simulink model "sim_model"  (R2021b)
settings: Solver=VariableStepAuto  StartTime=0.0  StopTime=10.0  RelTol=1e-3
settings Model: Creator=matteodepaola  LastModifiedBy=matteodepaola

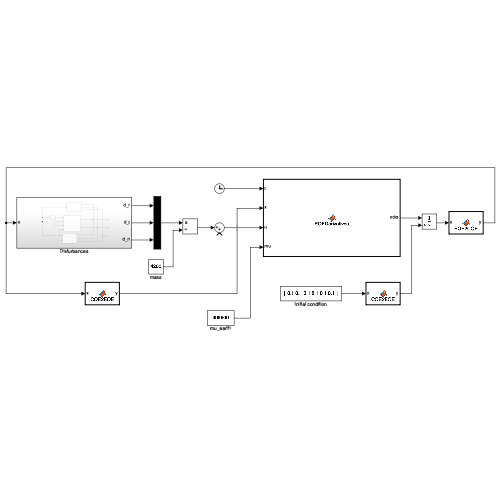
[thumbnail: Simulink's stored preview of the top-level diagram]
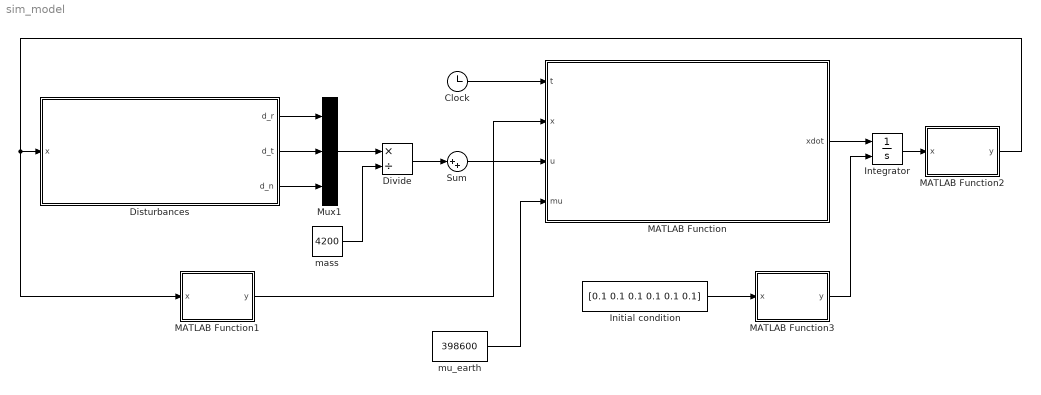
== system sim_model ==
  Clock : Clock
  Disturbances : Subsystem
  Divide : Product  Inputs=*/
  Initial condition : Constant  Value=[0.1 0.1 0.1 0.1 0.1 0.1]
  Integrator : Integrator  InitialConditionSource=external
  MATLAB Function : MATLAB Function  TreatAsAtomicUnit=on
  MATLAB Function1 : MATLAB Function  TreatAsAtomicUnit=on
  MATLAB Function2 : MATLAB Function  TreatAsAtomicUnit=on
  MATLAB Function3 : MATLAB Function  TreatAsAtomicUnit=on
  Mux1 : Mux  Inputs=3
  Sum : Sum  Inputs=|++
  mass : Constant  Value=4200
  mu_earth : Constant  Value=398600
  wires:
  MATLAB Function/1(xdot) -> Integrator/1
  MATLAB Function1/1(y) -> MATLAB Function/2(x)
  Clock/1 -> MATLAB Function/1(t)
  mu_earth/1 -> MATLAB Function/4(mu)
  Disturbances/1(d_r) -> Mux1/1
  Disturbances/2(d_t) -> Mux1/2
  Disturbances/3(d_n) -> Mux1/3
  Sum/1 -> MATLAB Function/3(u)
  mass/1 -> Divide/2
  Mux1/1 -> Divide/1
  Divide/1 -> Sum/1
  Integrator/1 -> MATLAB Function2/1(x)
  MATLAB Function2/1(y) -> MATLAB Function1/1(x), Disturbances/1(x)
  Initial condition/1 -> MATLAB Function3/1(x)
  MATLAB Function3/1(y) -> Integrator/2

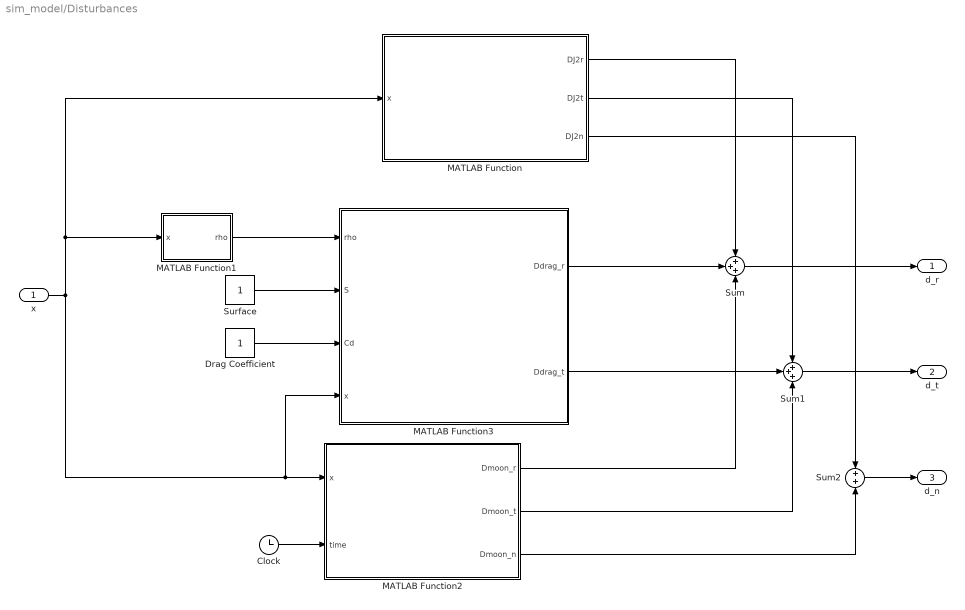
== system sim_model/Disturbances ==
  x : Inport
  Clock : Clock
  Drag Coefficient : Constant
  MATLAB Function : MATLAB Function  TreatAsAtomicUnit=on
  MATLAB Function1 : MATLAB Function  TreatAsAtomicUnit=on
  MATLAB Function2 : MATLAB Function  TreatAsAtomicUnit=on
  MATLAB Function3 : MATLAB Function  TreatAsAtomicUnit=on
  Sum : Sum  Inputs=+++
  Sum1 : Sum  Inputs=+++
  Sum2 : Sum  Inputs=+|+
  Surface : Constant
  d_r : Outport
  d_t : Outport  Port=2
  d_n : Outport  Port=3
  wires:
  MATLAB Function/3(DJ2n) -> Sum2/1
  x/1 -> MATLAB Function/1(x), MATLAB Function1/1(x), MATLAB Function3/4(x), MATLAB Function2/1(x)
  MATLAB Function/1(DJ2r) -> Sum/1
  MATLAB Function1/1(rho) -> MATLAB Function3/1(rho)
  Clock/1 -> MATLAB Function2/2(time)
  Drag Coefficient/1 -> MATLAB Function3/3(Cd)
  MATLAB Function3/1(Ddrag_r) -> Sum/2
  Surface/1 -> MATLAB Function3/2(S)
  MATLAB Function2/1(Dmoon_r) -> Sum/3
  MATLAB Function/2(DJ2t) -> Sum1/1
  MATLAB Function3/2(Ddrag_t) -> Sum1/2
  MATLAB Function2/2(Dmoon_t) -> Sum1/3
  MATLAB Function2/3(Dmoon_n) -> Sum2/2
  Sum/1 -> d_r/1
  Sum1/1 -> d_t/1
  Sum2/1 -> d_n/1

== matlab function sim_model/Disturbances/MATLAB Function1 ==
  data: x input; rho output
function rho = rho_selection(x)
a = x(1);
e = x(2);
theta = x(6);

% [km kg/m^3 km] % check Bernelli slides for references
rho_table = [0 1.225 7.249 ;
    25 3.899e-2 6.349 ;
    30 1.774e-2 6.682 ;
    40 3.972e-3 7.554 ;
    50 1.057e-3 8.382 ;
    60 3.206e-4 7.714 ;
    70 8.770e-5 6.549 ;
    80 1.905e-5 5.779 ;
    90 3.396e-6 5.382 ;
    100 5.297e-7 5.877 ;
    110 9.661e-8 7.263 ;
    120 2.438e-8 9.473 ;
    130 8.484e-9 12.636 ;
    140 3.845e-9 16.149 ;
    150 2.070e-9 22.523 ;
    180 5.464e-10 29.740 ;
    200 2.789e-10 37.105 ;
    250 7.248e-11 45.548 ;
    300 2.418e-11 53.628 ;
    350 9.158e-12 53.298 ;
    400 3.725e-12 58.515 ;
    450 1.585e-12 60.828 ;
    500 6.967e-13 63.822 ;
    600 1.454e-13 71.835 ;
    700 3.614e-14 88.667 ;
    800 1.170e-14 124.64 ;
    900 5.245e-15 181.05 ;
    1000 3.019e-15 268.00];


p = a*(1-e^2); % semilatum rectum [km]
r = p/(1+e*cos(theta)); % distance from focus in km
earth_radius = 6.3781e+3; %[km] %correction, before it was e+6
h = r - earth_radius; %[km]
% R = sqrt(r^2+(e*a)^2+2*r*e*a*cos(theta)) % distance from earth

%selection of rho_
select = 0;

for ind = 2:28
    if h < rho_table(ind,1)
        select = ind - 1;
        break
    end
end

if select == 0
    select = 28;
end

h_0     =   rho_table(select, 1);
rho_0   =   rho_table(select, 2);
H       =   rho_table(select, 3);
rho = rho_0*exp(-(h-h_0)/H);

== matlab function sim_model/Disturbances/MATLAB Function ==
  data: x input; DJ2r output; DJ2t output; DJ2n output
function[DJ2r, DJ2t, DJ2n] = earthNonSphericity(x)

J2 = 0.001082;  % geopotential coefficient of earth's oblateness
mu_earth = 398600;    % [km^3*s^-3] standard gravitational parameter of earh (mu = G*M)
Re = 6371;      % [km] earth equatorial radius

a = x(1);
e = x(2);
i = x(3);
Omega = x(4);
w = x(5);
theta = x(6);

h = cos(OM)*tan(i/2);
k = sin(OM)*tan(i/2);
L = OM+om+theta;

[rr,~] = paraorb2rv(a,e,i,Omega,w,theta,mu_earth);

r = sqrt(rr(1)^2+rr(2)^2+rr(3)^2);

DJ2r = -(3*mu_earth*J2*Re^2)/(2*r^4)*(1-12*(h*sin(L)-k*cos(L)^2)/(1+h^2+k^2)^2);
DJ2t = -(12*mu_earth*J2*Re^2)/(r^4)*(h*sin(L)-k*cos(L))*(h*cos(L)+k*sin(L))/(1+h^2+k^2)^2;
DJ2n = -(6*mu_earth*J2*Re^2)/(r^4)*(1-h^2-k^2)*(h*sin(L)-k*cos(L))/(1+h^2+k^2)^2;

== matlab function sim_model/Disturbances/MATLAB Function2 ==
  data: x input; Dmoon_r output; time input; Dmoon_t output; Dmoon_n output
function [Dmoon_r, Dmoon_t, Dmoon_n]  = moonDisturbance(x,time)

a = x(1);
e = x(2);
i = x(3);
Omega = x(4);
w = x(5);
theta = x(6);

mu_earth = 398600;
[r,v] = paraorb2rv(a,e,i,Omega,w,theta,mu_earth);

c = 2459945.50000; % Julian day for 1/1/2023 at 00:00:00

time = time/86400 + c; % from seconds to Julian day in TDT scale
% r position vector of the spacecraft
% time is the value representing the Julian day in TDT scale

mu_moon = 490487;               % moon standard gravitational coefficient

cd ./'Moon Position'/
[x_m, y_m, z_m] = moonpos(time);
cd ../
s = [x_m y_m z_m]';


d = r-s;                            % vector from moon to spacecraft
d_mod = sqrt(d(1)^2+d(2)^2+d(3)^2); % modulus of d
q = r'*(r-2*s)/(s'*s);
F = @(q) q*(3+3*q+q^2)/(1+(1+q)^(3/2));

t = -mu_moon/d_mod^3*(r+F(q)*s);

ir = r/norm(r);
in = cross(r,v)/norm(cross(r,v));
it = cross(in,ir);

Q = [ir it in];

a_tb = Q*t;

Dmoon_r = a_tb(1);
Dmoon_t = a_tb(2);
Dmoon_n = a_tb(3);

== matlab function sim_model/Disturbances/MATLAB Function3 ==
  data: rho input; Ddrag_r output; S input; Cd input; x input; Ddrag_t output
function [Ddrag_r, Ddrag_t] = drag(rho,S,Cd,x)

a = x(1);
e = x(2);
i = x(3);
Omega = x(4);
w = x(5);
theta = x(6);

mu_earth = 398600;
[~,vv] = paraorb2rv(a,e,i,Omega,w,theta,mu_earth);

p = a*(1-e^2);
f = e*cos(w+Omega);
g = e*sin(w+Omega);
% h = cos(Omega)*tan(i/2);
% k = sin(Omega)*tan(i/2);
L = Omega+w+theta;


v_mod = sqrt(vv(1)^2+vv(2)^2+vv(3)^2);
v_r   = sqrt(mu_earth/p)*(f*sin(L)-g*cos(L));
v_t   = sqrt(mu_earth/p)*(1+f*cos(L)+g*sin(L));

Ddrag_r = -1/2*rho*S*Cd*v_mod*v_r;
Ddrag_t = -1/2*rho*S*Cd*v_mod*v_t;
end

== matlab function sim_model/MATLAB Function ==
  data: t input; x input; u input; xdot output; mu input
function xdot = EOEDerivatives(t, x, u, mu)

% Equinoctial Orbital Elements
p = x(1);
if p < 0
    p = -p;
%     warning('p became negative. Switched to absolute value for calculations');
end
f = x(2);
g = x(3);
h = x(4);
k = x(5);
L = x(6);

% Accelerations
ar = u(1);
at = u(2);
an = u(3);

% Definition of useful values
w = 1 + f*cos(L)+g*sin(L);
% r = p/w;
s2 = 1+h^2+k^2;
% alpha2 = h^2-k^2;
p_mu05 = sqrt(p/mu);

% State Derivative Calculation
pdot = 2*p/w*p_mu05*at;
fdot = p_mu05*(ar*sin(L) + ((w+1)*cos(L)+f)*at/w - (h*sin(L)-k*cos(L))*g*an/w);
gdot = p_mu05*(-ar*cos(L) + ((w+1)*sin(L)+g)*at/w + (h*sin(L)-k*cos(L))*g*an/w);
hdot = p_mu05*s2*an/2/w*cos(L);
kdot = p_mu05*s2*an/2/w*sin(L);
Ldot = sqrt(mu*p)*(w/p)^2+p_mu05/w*(h*sin(L)-k*cos(L))*an;

xdot = [pdot fdot gdot hdot kdot Ldot]';

== matlab function sim_model/MATLAB Function1 ==
  data: x input; y output
function y  = COE2EOE(x)

%COE2EOE  Function to convert Classical Orbital Elements to Equinoctial 
%   Orbital Elements.
%   EOE = COE2EOE(COE) receives as input a vector of the 6 classical OE and
%   gives as output a column vector of the 6 equinoctial OE.
%   In particular, the input vector must be of the form 
%   COE = [a e i om OM theta], where
%       a: semimajor axis
%       e: eccentricity
%       i: inclination
%       om: argument of periapsis
%       OM: longitude of the ascending node
%       theta: true anomaly
%   The output vector is in the form EOE = [p f g h k L], where p is the 
%   semilatus rectum and L is the true longitude

if isa(x, 'double')

    a = x(1);
    e = x(2);
    i = x(3);
    OM = x(4);
    om = x(5);
    theta = x(6);

elseif isa(x, 'struct')

    a = x.a;
    e = x.e;
    i = x.i;
    om = x.om;
    OM = x.OM;
    theta = x.theta;

end  

p = a*(1-e^2);
f = e*cos(om+OM);
g = e*sin(om+OM);
h = cos(OM)*tan(i/2);
k = sin(OM)*tan(i/2);
L = OM+om+theta;

y = [p f g h k L]';

== matlab function sim_model/MATLAB Function2 ==
  data: x input; y output
function y  = EOE2COE(x)

%EOE2COE  Function to convert Equinoctial Orbital Elements to Classical 
%   Orbital Elements.
%   COE = EOE2COE(EOE) receives as input a vector of the 6 equinoctial OE and
%   gives as output a column vector of the 6 classical OE.
%   In particular, the input vector must be of the form EOE = [p f g h k L],
%   where p is the semilatus rectum and L is the true longitude
%   The output vector is in the form COE = [a e i om OM theta]', where
%       a: semimajor axis
%       e: eccentricity
%       i: inclination
%       om: argument of periapsis
%       OM: longitude of the ascending node
%       theta: true anomaly

p = x(1);
f = x(2);
g = x(3);
h = x(4);
k = x(5);
L = x(6);

a = p/(1-f^2-g^2);
e = sqrt(f^2+g^2);
i = atan2(2*sqrt(h^2+k^2), 1-h^2-k^2);
OM = atan2(k,h);
om = atan2(g*h-f*k, f*h+g*k);
theta = L-OM-om;

y = [a e i OM om theta]';

% u = om+theta Argument of latitude

== matlab function sim_model/MATLAB Function3 ==
  data: x input; y output
function y  = COE2EOE(x)

%COE2EOE  Function to convert Classical Orbital Elements to Equinoctial 
%   Orbital Elements.
%   EOE = COE2EOE(COE) receives as input a vector of the 6 classical OE and
%   gives as output a column vector of the 6 equinoctial OE.
%   In particular, the input vector must be of the form 
%   COE = [a e i om OM theta], where
%       a: semimajor axis
%       e: eccentricity
%       i: inclination
%       om: argument of periapsis
%       OM: longitude of the ascending node
%       theta: true anomaly
%   The output vector is in the form EOE = [p f g h k L], where p is the 
%   semilatus rectum and L is the true longitude

if isa(x, 'double')

    a = x(1);
    e = x(2);
    i = x(3);
    OM = x(4);
    om = x(5);
    theta = x(6);

elseif isa(x, 'struct')

    a = x.a;
    e = x.e;
    i = x.i;
    om = x.om;
    OM = x.OM;
    theta = x.theta;

end  

p = a*(1-e^2);
f = e*cos(om+OM);
g = e*sin(om+OM);
h = cos(OM)*tan(i/2);
k = sin(OM)*tan(i/2);
L = OM+om+theta;

y = [p f g h k L]';
